simulink model "week2_que3"  (R2020b)
settings: Solver=ode45  StartTime=0.0  StopTime=120  RelTol=1e-3
model workspace (MAT data in the model file):
  b = 50
  m = 1000
settings Model: DataDictionary=Cruisecontrol_q3.sldd  Creator=mluser  LastModifiedBy=mluser

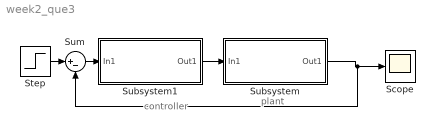
== system week2_que3 ==
  note: plant
  note: controller
  Scope : Scope
  Step : Step  Time=0  After=500  SampleTime=0
  Subsystem : Subsystem
  Subsystem1 : Subsystem
  Sum : Sum  Inputs=|+-
  wires:
  Subsystem/1(Out1) -> Sum/2, Scope/1
  Step/1 -> Sum/1
  Subsystem1/1(Out1) -> Subsystem/1(In1)
  Sum/1 -> Subsystem1/1(In1)

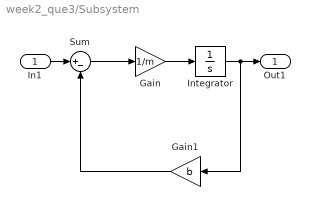
== system week2_que3/Subsystem ==
  In1 : Inport
  Gain : Gain  Gain=1/m
  Gain1 : Gain  Gain=b
  Integrator : Integrator
  Sum : Sum  Inputs=|+-
  Out1 : Outport
  wires:
  Integrator/1 -> Out1/1, Gain1/1
  Gain/1 -> Integrator/1
  Gain1/1 -> Sum/2
  Sum/1 -> Gain/1
  In1/1 -> Sum/1

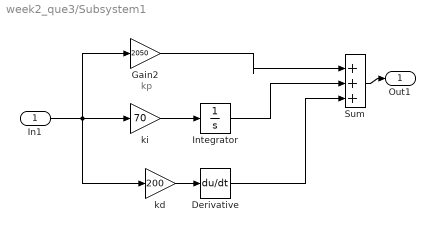
== system week2_que3/Subsystem1 ==
  note: kp
  In1 : Inport
  Derivative : Derivative
  Gain2 : Gain  Gain=2050
  Integrator : Integrator
  Sum : Sum  Inputs=|+++
  kd : Gain  Gain=200
  ki : Gain  Gain=70
  Out1 : Outport
  wires:
  kd/1 -> Derivative/1
  In1/1 -> kd/1, Gain2/1, ki/1
  Gain2/1 -> Sum/1
  ki/1 -> Integrator/1
  Integrator/1 -> Sum/2
  Derivative/1 -> Sum/3
  Sum/1 -> Out1/1
